simulink model "Pendulolnvertido"  (R2017b)
settings: Solver=ode4  StartTime=0.0  StopTime=30.0  RelTol=1e-3
undefined symbols (not defined in the file): b, g, I, l, m, M
settings Model: Creator=Benjamin Nicolas  LastModifiedBy=Benjamin Nicolas

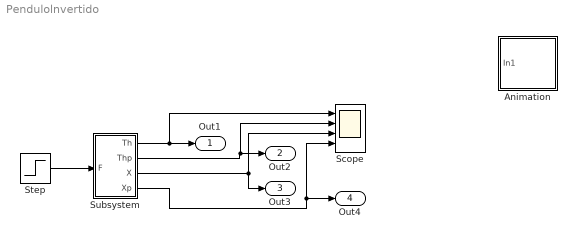
== system Pendulolnvertido ==
  Animation : Subsystem  mask(Pendulum plot){RefBlock=Initial, doAnimation=false}
      mask prompts: RefBlock "DC reference signal block name:"; doAnimation "Show animation"
      mask help: Pendulum plot
      mask Help: Pendulum animation function using Handle graphics.
      mask Display: plot([-10 10],[0 0],[-2 -2 2 2],[0 1 1 0],[0 3],[1 5])
  Scope : Scope  NumInputPorts=4
  Step : Step  SampleTime=0
  Subsystem : Subsystem
  Out1 : Outport
  Out2 : Outport  Port=2
  Out3 : Outport  Port=3
  Out4 : Outport  Port=4
  wires:
  Subsystem/1("Th ") -> Out1/1, Scope/1
  Subsystem/2("Thp ") -> Scope/2, Out2/1
  Subsystem/3(X) -> Scope/3, Out3/1
  Subsystem/4("Xp ") -> Scope/4, Out4/1
  Step/1 -> Subsystem/1(F)

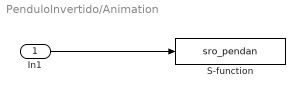
== system Pendulolnvertido/Animation ==
  In1 : Inport
  S-function : S-Function  FunctionName=sro_pendan  Parameters=RefBlock, doAnimation  SFunctionDeploymentMode=off  EnableBusSupport=off
      settings: DeleteFcn=sro_pendan([],[],[],'DeleteBlock');
  wires:
  In1/1 -> S-function/1

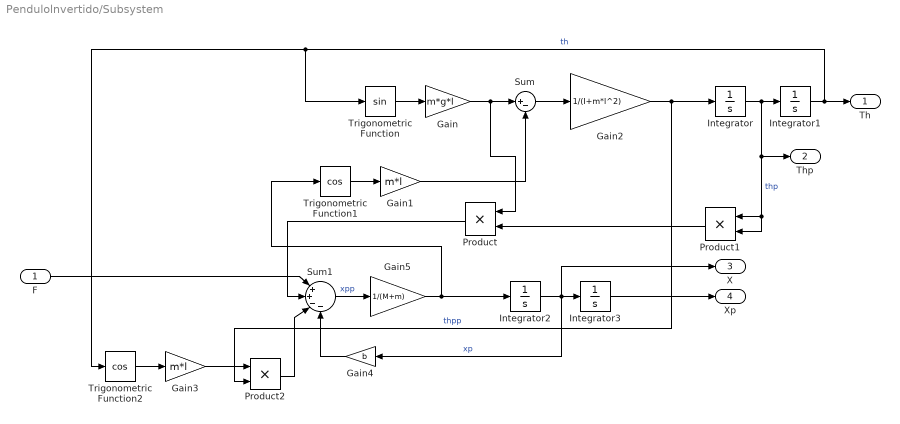
== system Pendulolnvertido/Subsystem ==
  F : Inport
  Gain : Gain  Gain=m*g*l
  Gain1 : Gain  Gain=m*l
  Gain2 : Gain  Gain=1/(I+m*l^2)
  Gain3 : Gain  Gain=m*l
  Gain4 : Gain  Gain=b
  Gain5 : Gain  Gain=1/(M+m)
  Integrator{,1..3} (4 alike) : Integrator  InitialCondition=1
  Product : Product
  Product1 : Product
  Product2 : Product
  Sum : Sum  Inputs=|+-
  Sum1 : Sum  Inputs=|++--
  Trigonometric Function : Trigonometry
  Trigonometric Function1 : Trigonometry  Operator=cos
  Trigonometric Function2 : Trigonometry  Operator=cos
  "Th " : Outport
  "Thp " : Outport  Port=2
  X : Outport  Port=3
  "Xp " : Outport  Port=4
  wires:
  Integrator3/1 -> "Xp "/1
  Gain/1 -> Product/1, Sum/1
  Trigonometric Function/1 -> Gain/1
  Sum/1 -> Gain2/1
  Gain2/1 -> Product2/2, Integrator/1  "thpp"
  Gain1/1 -> Sum/2
  Integrator1/1 -> "Th "/1, Trigonometric Function/1, Trigonometric Function2/1  "th"
  Trigonometric Function1/1 -> Gain1/1
  Gain3/1 -> Product2/1
  Product2/1 -> Sum1/3
  Integrator/1 -> "Thp "/1, Product1/2, Product1/1, Integrator1/1  "thp"
  Product/1 -> Sum1/2
  Gain4/1 -> Sum1/4
  Trigonometric Function2/1 -> Gain3/1
  F/1 -> Sum1/1
  Integrator2/1 -> X/1, Gain4/1, Integrator3/1  "xp"
  Sum1/1 -> Gain5/1  "xpp"
  Gain5/1 -> Integrator2/1, Trigonometric Function1/1
  Product1/1 -> Product/2
